simulink model "PubSub_Control_Thruster"  (R2018a)
settings: Solver=VariableStepAuto  StartTime=0.0  StopTime=inf  RelTol=1e-3
undefined symbols (not defined in the file or in its folder): angle_p_kp, angle_r_kp, angle_y_kp, Binv, Cx, Cy, DiscIntNeverNeededParam, Mx, My, omega_p_ki, omega_p_kp, omega_r_ki, omega_r_kp, omega_y_ki, omega_y_kp, RoboPlus_f2v_n, RoboPlus_f2v_p, Seabotix_f2v_n, Seabotix_f2v_p, serial, vx_kd, vx_ki, vx_kp, vy_kd, vy_ki, vy_kp, vz_ki, vz_kp, z_kp
libraries: simulink x10, robotlib x6, instrumentlib x2
settings Model: Creator=F.Takuya  LastModifiedBy=F.Takuya

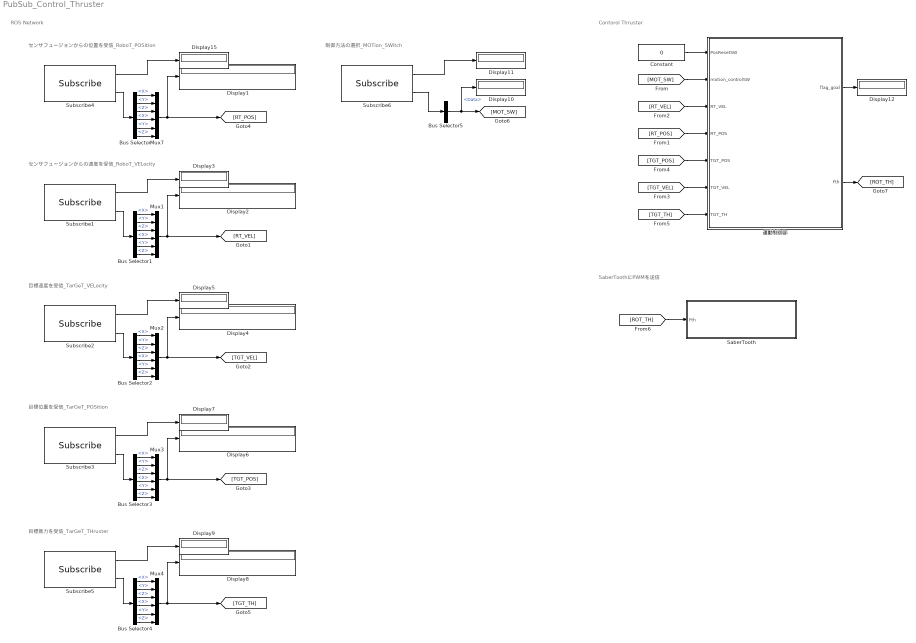
== system PubSub_Control_Thruster ==
  note: SaberToothにPWMを送信
  note: ROS Network
  note: センサフュージョンからの位置を受信_RoboT_POSition
  note: センサフュージョンからの速度を受信_RoboT_VELocity
  note: 目標速度を受信_TarGeT_VELocity
  note: 目標位置を受信_TarGeT_POSition
  note: 目標推力を受信_TarGeT_THruster
  note: 制御方法の選択_MOTion_SWitch
  note: Contorol Thruster
  Bus Selector{,1..4} (5 alike) : BusSelector  OutputSignals=Twist.Linear.X,Twist.Linear.Y,Twist.Linear.Z,Twist.Angular.X,Twist.Angular.Y,Twist.Angular.Z
  Bus Selector5 : BusSelector  OutputSignals=Data
  Constant : Constant  Value=0
  Display{1..12,15} (13 alike) : Display
  Mux{1..4,7} (5 alike) : Mux  Inputs=6
  SaberTooth : Subsystem
  Subscribe1 : robotlib/Subscribe  SourceLibraryInfo=This block requires Robotics System Toolbox  topicSource=Specify your own  topic=/RT_VEL  messageType=geometry_msgs/TwistStamped  sampleTime=-1  messageQueueLength=1
      settings: SourceProductBaseCode=RO
  Subscribe2 : robotlib/Subscribe  SourceLibraryInfo=This block requires Robotics System Toolbox  topicSource=Specify your own  topic=/TGT_VEL  messageType=geometry_msgs/TwistStamped  sampleTime=-1  messageQueueLength=1
      settings: SourceProductBaseCode=RO
  Subscribe3 : robotlib/Subscribe  SourceLibraryInfo=This block requires Robotics System Toolbox  topicSource=Specify your own  topic=/TGT_POS  messageType=geometry_msgs/TwistStamped  sampleTime=-1  messageQueueLength=1
      settings: SourceProductBaseCode=RO
  Subscribe4 : robotlib/Subscribe  SourceLibraryInfo=This block requires Robotics System Toolbox  topicSource=Specify your own  topic=/RT_POS  messageType=geometry_msgs/TwistStamped  sampleTime=-1  messageQueueLength=1
      settings: SourceProductBaseCode=RO
  Subscribe5 : robotlib/Subscribe  SourceLibraryInfo=This block requires Robotics System Toolbox  topicSource=Specify your own  topic=/TGT_TH  messageType=geometry_msgs/TwistStamped  sampleTime=-1  messageQueueLength=1
      settings: SourceProductBaseCode=RO
  Subscribe6 : robotlib/Subscribe  SourceLibraryInfo=This block requires Robotics System Toolbox  topicSource=Specify your own  topic=/MOT_SW  messageType=std_msgs/Float64  sampleTime=-1  messageQueueLength=1
      settings: SourceProductBaseCode=RO
  運動制御部 : Subsystem
  wires:
  Mux7/1 -> Display1/1, [RT_POS]
  Subscribe4/1 -> Display15/1
  Subscribe4/2 -> Bus Selector/1
  Bus Selector/1 -> Mux7/1  "<X>"
  Bus Selector/2 -> Mux7/2  "<Y>"
  Bus Selector/3 -> Mux7/3  "<Z>"
  Bus Selector/4 -> Mux7/4  "<X>"
  Bus Selector/5 -> Mux7/5  "<Y>"
  Bus Selector/6 -> Mux7/6  "<Z>"
  Subscribe1/2 -> Bus Selector1/1
  Bus Selector1/2 -> Mux1/2  "<Y>"
  Bus Selector1/1 -> Mux1/1  "<X>"
  Bus Selector1/5 -> Mux1/5  "<Y>"
  Mux1/1 -> Display2/1, [RT_VEL]
  Subscribe1/1 -> Display3/1
  Bus Selector1/4 -> Mux1/4  "<X>"
  Bus Selector1/3 -> Mux1/3  "<Z>"
  Bus Selector1/6 -> Mux1/6  "<Z>"
  Bus Selector2/3 -> Mux2/3  "<Z>"
  Subscribe2/1 -> Display5/1
  Bus Selector2/4 -> Mux2/4  "<X>"
  Bus Selector2/6 -> Mux2/6  "<Z>"
  Mux2/1 -> Display4/1, [TGT_VEL]
  Bus Selector2/5 -> Mux2/5  "<Y>"
  Bus Selector2/2 -> Mux2/2  "<Y>"
  Subscribe2/2 -> Bus Selector2/1
  Bus Selector2/1 -> Mux2/1  "<X>"
  Bus Selector3/4 -> Mux3/4  "<X>"
  Mux3/1 -> Display6/1, [TGT_POS]
  Bus Selector3/2 -> Mux3/2  "<Y>"
  Bus Selector3/1 -> Mux3/1  "<X>"
  Bus Selector3/5 -> Mux3/5  "<Y>"
  Bus Selector3/3 -> Mux3/3  "<Z>"
  Subscribe3/1 -> Display7/1
  Bus Selector3/6 -> Mux3/6  "<Z>"
  Subscribe3/2 -> Bus Selector3/1
  Subscribe5/2 -> Bus Selector4/1
  Subscribe5/1 -> Display9/1
  Bus Selector4/1 -> Mux4/1  "<X>"
  Bus Selector4/2 -> Mux4/2  "<Y>"
  Bus Selector4/6 -> Mux4/6  "<Z>"
  Bus Selector4/3 -> Mux4/3  "<Z>"
  Bus Selector4/4 -> Mux4/4  "<X>"
  Mux4/1 -> Display8/1, [TGT_TH]
  Bus Selector4/5 -> Mux4/5  "<Y>"
  Subscribe6/1 -> Display11/1
  Subscribe6/2 -> Bus Selector5/1
  Bus Selector5/1 -> Display10/1, [MOT_SW]  "<Data>"
  [TGT_TH] -> 運動制御部/7(TGT_TH)
  [TGT_VEL] -> 運動制御部/6(TGT_VEL)
  [TGT_POS] -> 運動制御部/5(TGT_POS)
  [RT_POS] -> 運動制御部/4(RT_POS)
  [RT_VEL] -> 運動制御部/3(RT_VEL)
  [MOT_SW] -> 運動制御部/2(motion_controlSW)
  運動制御部/2(Fth) -> [ROT_TH]
  運動制御部/1(flag_goal) -> Display12/1
  Constant/1 -> 運動制御部/1(PosResetSW)
  [ROT_TH] -> SaberTooth/1(Fth)

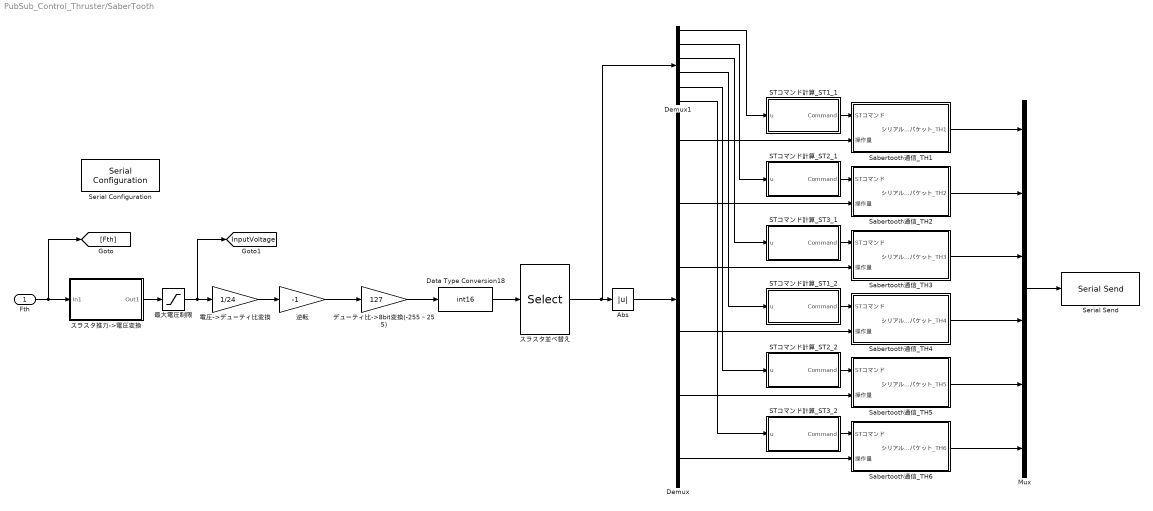
== system PubSub_Control_Thruster/SaberTooth ==
  Fth : Inport
  Abs : Abs
  Data Type Conversion18 : DataTypeConversion  OutDataTypeStr=int16
  Demux : Demux  Outputs=6
  Demux1 : Demux  Outputs=6
  Mux : Mux  Inputs=6
  STコマンド計算_ST1_1 : MATLAB Function  TreatAsAtomicUnit=on
  STコマンド計算_ST1_2 : MATLAB Function  TreatAsAtomicUnit=on
  STコマンド計算_ST2_1 : MATLAB Function  TreatAsAtomicUnit=on
  STコマンド計算_ST2_2 : MATLAB Function  TreatAsAtomicUnit=on
  STコマンド計算_ST3_1 : MATLAB Function  TreatAsAtomicUnit=on
  STコマンド計算_ST3_2 : MATLAB Function  TreatAsAtomicUnit=on
  Sabertooth通信_TH1 : Subsystem
  Sabertooth通信_TH2 : Subsystem
  Sabertooth通信_TH3 : Subsystem
  Sabertooth通信_TH4 : Subsystem
  Sabertooth通信_TH5 : Subsystem
  Sabertooth通信_TH6 : Subsystem
  Serial Configuration : instrumentlib/Serial Configuration  Priority=-200000  ComPortMenu=<Please select a port...>  ComPort=COM9  ObjConstructor=serial('COM9');  BaudRate=9600  DataBits=8  Parity=none  StopBits=1  FlowControl=none  Timeout=10  ByteOrder=LittleEndian
  Serial Send : instrumentlib/Serial Send  ComPortMenu=<Please select a port...>  ComPort=COM9  ObjConstructor=serial('COM9');  Terminator=<none>  EnableBlockingMode=on
  スラスタ並べ替え : Selector  InputPortWidth=6  IndexOptions=Index vector (dialog)  Indices=[4 5 1 6 3 2]  OutputSizes=1
  スラスタ推力->電圧変換 : Subsystem
  デューティ比->8bit変換(-255～255) : Gain  Gain=127
  最大電圧制限 : Saturate  UpperLimit=24  LowerLimit=-24
  逆転 : Gain  Gain=-1
  電圧->デューティ比変換 : Gain  Gain=1/24
  tag scope: InputVoltage=global
  wires:
  電圧->デューティ比変換/1 -> 逆転/1
  スラスタ推力->電圧変換/1(Out1) -> 最大電圧制限/1
  Fth/1 -> [Fth], スラスタ推力->電圧変換/1(In1)
  STコマンド計算_ST3_2/1(Command) -> Sabertooth通信_TH6/1(STコマンド)
  Sabertooth通信_TH4/1(シリアルパケット_TH4) -> Mux/4
  STコマンド計算_ST1_1/1(Command) -> Sabertooth通信_TH1/1(STコマンド)
  Sabertooth通信_TH1/1(シリアルパケット_TH1) -> Mux/1
  Mux/1 -> Serial Send/1
  Demux/3 -> Sabertooth通信_TH3/2(操作量)
  Sabertooth通信_TH5/1(シリアルパケット_TH5) -> Mux/5
  Demux/4 -> Sabertooth通信_TH4/2(操作量)
  Sabertooth通信_TH2/1(シリアルパケット_TH2) -> Mux/2
  Sabertooth通信_TH3/1(シリアルパケット_TH3) -> Mux/3
  Demux/1 -> Sabertooth通信_TH1/2(操作量)
  Sabertooth通信_TH6/1(シリアルパケット_TH6) -> Mux/6
  Demux/2 -> Sabertooth通信_TH2/2(操作量)
  Abs/1 -> Demux/1
  Demux/5 -> Sabertooth通信_TH5/2(操作量)
  Demux/6 -> Sabertooth通信_TH6/2(操作量)
  STコマンド計算_ST2_1/1(Command) -> Sabertooth通信_TH2/1(STコマンド)
  STコマンド計算_ST2_2/1(Command) -> Sabertooth通信_TH5/1(STコマンド)
  STコマンド計算_ST1_2/1(Command) -> Sabertooth通信_TH4/1(STコマンド)
  STコマンド計算_ST3_1/1(Command) -> Sabertooth通信_TH3/1(STコマンド)
  Demux1/6 -> STコマンド計算_ST3_2/1(u)
  Demux1/5 -> STコマンド計算_ST2_2/1(u)
  Demux1/4 -> STコマンド計算_ST1_2/1(u)
  Demux1/3 -> STコマンド計算_ST3_1/1(u)
  Demux1/2 -> STコマンド計算_ST2_1/1(u)
  Demux1/1 -> STコマンド計算_ST1_1/1(u)
  デューティ比->8bit変換(-255～255)/1 -> Data Type Conversion18/1
  Data Type Conversion18/1 -> スラスタ並べ替え/1
  スラスタ並べ替え/1 -> Abs/1, Demux1/1
  最大電圧制限/1 -> [InputVoltage], 電圧->デューティ比変換/1
  逆転/1 -> デューティ比->8bit変換(-255～255)/1

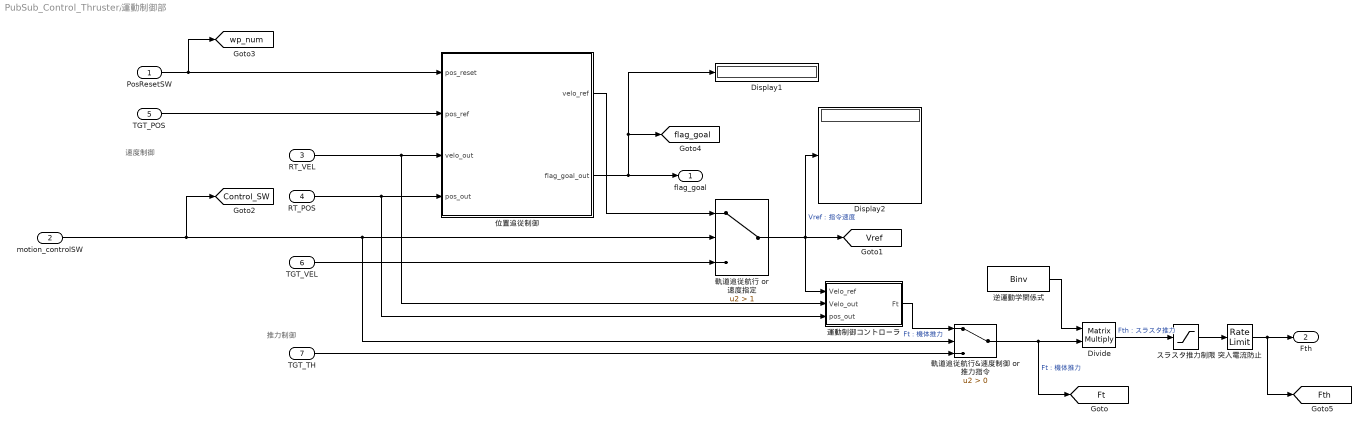
== system PubSub_Control_Thruster/運動制御部 ==
  note: 推力制御
  note: 速度制御
  PosResetSW : Inport
  motion_controlSW : Inport  Port=2
  RT_VEL : Inport  Port=3
  RT_POS : Inport  Port=4
  TGT_POS : Inport  Port=5
  TGT_VEL : Inport  Port=6
  TGT_TH : Inport  Port=7
  Display1 : Display
  Display2 : Display
  Divide : Product  Inputs=**  Multiplication=Matrix(*)
  スラスタ推力制限 : Saturate  UpperLimit=20  LowerLimit=-20
  位置追従制御 : Stateflow chart  TreatAsAtomicUnit=on
  突入電流防止 : RateLimiter  RisingSlewLimit=50  FallingSlewLimit=-50  SampleTimeMode=inherited
  軌道追従航行 or 速度指定 : Switch  Criteria=u2 > Threshold  Threshold=1
  軌道追従航行&速度制御 or 推力指令 : Switch  Criteria=u2 > Threshold
  逆運動学関係式 : Constant  Value=Binv
  運動制御コントローラ : Subsystem
  flag_goal : Outport
  Fth : Outport  Port=2
  tag scope: Control_SW=global, Ft=global, Fth=global, Vref=global, flag_goal=global, wp_num=global
  wires:
  軌道追従航行&速度制御 or 推力指令/1 -> [Ft], Divide/2  "Ft : 機体推力"
  軌道追従航行 or 速度指定/1 -> 運動制御コントローラ/1(Velo_ref), Display2/1, [Vref]  "Vref : 指令速度"
  逆運動学関係式/1 -> Divide/1
  Divide/1 -> スラスタ推力制限/1  "Fth : スラスタ推力"
  motion_controlSW/1 -> [Control_SW], 軌道追従航行&速度制御 or 推力指令/2, 軌道追従航行 or 速度指定/2
  TGT_VEL/1 -> 軌道追従航行 or 速度指定/3
  RT_VEL/1 -> 運動制御コントローラ/2(Velo_out), 位置追従制御/3(velo_out)
  運動制御コントローラ/1(Ft) -> 軌道追従航行&速度制御 or 推力指令/1  "Ft : 機体推力"
  RT_POS/1 -> 運動制御コントローラ/3(pos_out), 位置追従制御/4(pos_out)
  PosResetSW/1 -> 位置追従制御/1(pos_reset), [wp_num]
  位置追従制御/1(velo_ref) -> 軌道追従航行 or 速度指定/1
  TGT_TH/1 -> 軌道追従航行&速度制御 or 推力指令/3
  スラスタ推力制限/1 -> 突入電流防止/1
  突入電流防止/1 -> [Fth], Fth/1
  位置追従制御/2(flag_goal_out) -> Display1/1, [flag_goal], flag_goal/1
  TGT_POS/1 -> 位置追従制御/2(pos_ref)

== system PubSub_Control_Thruster/SaberTooth/Sabertooth通信_TH1 ==
  STコマンド : Inport
  操作量 : Inport  Port=2
  Add : Sum  Inputs=+++
  Address : Constant  Value=128  OutDataTypeStr=uint8
  Bitwise Operator : simulink/Logic and Bit Operations/Bitwise Operator  logicop=AND  UseBitMask=on  BitMask=bin2dec('01111111')  BitMaskRealWorld=Stored Integer
  Data Type Conversion{,1..3} (4 alike) : DataTypeConversion  OutDataTypeStr=uint8
  Mux : Mux
  Saturation : Saturate  UpperLimit=255  LowerLimit=0
  Saturation1 : Saturate  UpperLimit=255  LowerLimit=0
  Scope : Scope
  シリアルパケット_TH1 : Outport
  wires:
  Bitwise Operator/1 -> Mux/4  "チェックサム address byte  + command byte  + data byte"
  Data Type Conversion2/1 -> Saturation1/1
  Data Type Conversion1/1 -> Bitwise Operator/1
  STコマンド/1 -> Data Type Conversion3/1  "コマンド [モーター１] 0：正転　1：逆転 [モーター2] 4：正転　5：逆転"
  操作量/1 -> Data Type Conversion2/1
  Mux/1 -> Saturation/1
  Data Type Conversion/1 -> シリアルパケット_TH1/1
  Add/1 -> Data Type Conversion1/1
  Saturation/1 -> Data Type Conversion/1
  Address/1 -> Add/1, Mux/1  "Sabertoothのアドレス（どのSTと通信するか）"
  Saturation1/1 -> Scope/1, Add/3, Mux/3  "操作量(uint8の0～255)"
  Data Type Conversion3/1 -> Add/2, Mux/2

== system PubSub_Control_Thruster/SaberTooth/Sabertooth通信_TH2 ==
  STコマンド : Inport
  操作量 : Inport  Port=2
  Add : Sum  Inputs=+++
  Address : Constant  Value=129  OutDataTypeStr=uint8
  Bitwise Operator : simulink/Logic and Bit Operations/Bitwise Operator  logicop=AND  UseBitMask=on  BitMask=bin2dec('01111111')  BitMaskRealWorld=Stored Integer
  Data Type Conversion{,1..3} (4 alike) : DataTypeConversion  OutDataTypeStr=uint8
  Mux : Mux
  Saturation : Saturate  UpperLimit=255  LowerLimit=0
  Saturation1 : Saturate  UpperLimit=255  LowerLimit=0
  Scope : Scope
  シリアルパケット_TH2 : Outport
  wires:
  Bitwise Operator/1 -> Mux/4  "チェックサム address byte  + command byte  + data byte"
  Data Type Conversion2/1 -> Saturation1/1
  Data Type Conversion1/1 -> Bitwise Operator/1
  STコマンド/1 -> Data Type Conversion3/1  "コマンド [モーター１] 0：正転　1：逆転 [モーター2] 4：正転　5：逆転"
  操作量/1 -> Data Type Conversion2/1
  Mux/1 -> Saturation/1
  Data Type Conversion/1 -> シリアルパケット_TH2/1
  Add/1 -> Data Type Conversion1/1
  Saturation/1 -> Data Type Conversion/1
  Address/1 -> Add/1, Mux/1  "Sabertoothのアドレス（どのSTと通信するか）"
  Saturation1/1 -> Scope/1, Add/3, Mux/3  "操作量(uint8の0～255)"
  Data Type Conversion3/1 -> Add/2, Mux/2

== system PubSub_Control_Thruster/SaberTooth/Sabertooth通信_TH3 ==
  STコマンド : Inport
  操作量 : Inport  Port=2
  Add : Sum  Inputs=+++
  Address : Constant  Value=130  OutDataTypeStr=uint8
  Bitwise Operator : simulink/Logic and Bit Operations/Bitwise Operator  logicop=AND  UseBitMask=on  BitMask=bin2dec('01111111')  BitMaskRealWorld=Stored Integer
  Data Type Conversion{,1..3} (4 alike) : DataTypeConversion  OutDataTypeStr=uint8
  Mux : Mux
  Saturation : Saturate  UpperLimit=255  LowerLimit=0
  Saturation1 : Saturate  UpperLimit=255  LowerLimit=0
  Scope : Scope
  シリアルパケット_TH3 : Outport
  wires:
  Bitwise Operator/1 -> Mux/4  "チェックサム address byte  + command byte  + data byte"
  Data Type Conversion2/1 -> Saturation1/1
  Data Type Conversion1/1 -> Bitwise Operator/1
  STコマンド/1 -> Data Type Conversion3/1  "コマンド [モーター１] 0：正転　1：逆転 [モーター2] 4：正転　5：逆転"
  操作量/1 -> Data Type Conversion2/1
  Mux/1 -> Saturation/1
  Data Type Conversion/1 -> シリアルパケット_TH3/1
  Add/1 -> Data Type Conversion1/1
  Saturation/1 -> Data Type Conversion/1
  Address/1 -> Add/1, Mux/1  "Sabertoothのアドレス（どのSTと通信するか）"
  Saturation1/1 -> Scope/1, Add/3, Mux/3  "操作量(uint8の0～255)"
  Data Type Conversion3/1 -> Add/2, Mux/2

== system PubSub_Control_Thruster/SaberTooth/Sabertooth通信_TH4 ==
  STコマンド : Inport
  操作量 : Inport  Port=2
  Add : Sum  Inputs=+++
  Address : Constant  Value=128  OutDataTypeStr=uint8
  Bitwise Operator : simulink/Logic and Bit Operations/Bitwise Operator  logicop=AND  UseBitMask=on  BitMask=bin2dec('01111111')  BitMaskRealWorld=Stored Integer
  Data Type Conversion{,1..3} (4 alike) : DataTypeConversion  OutDataTypeStr=uint8
  Mux : Mux
  Saturation : Saturate  UpperLimit=255  LowerLimit=0
  Saturation1 : Saturate  UpperLimit=255  LowerLimit=0
  Scope : Scope
  シリアルパケット_TH4 : Outport
  wires:
  Bitwise Operator/1 -> Mux/4  "チェックサム address byte  + command byte  + data byte"
  Data Type Conversion2/1 -> Saturation1/1
  Data Type Conversion1/1 -> Bitwise Operator/1
  STコマンド/1 -> Data Type Conversion3/1  "コマンド [モーター１] 0：正転　1：逆転 [モーター2] 4：正転　5：逆転"
  操作量/1 -> Data Type Conversion2/1
  Mux/1 -> Saturation/1
  Data Type Conversion/1 -> シリアルパケット_TH4/1
  Add/1 -> Data Type Conversion1/1
  Saturation/1 -> Data Type Conversion/1
  Address/1 -> Add/1, Mux/1  "Sabertoothのアドレス（どのSTと通信するか）"
  Saturation1/1 -> Scope/1, Add/3, Mux/3  "操作量(uint8の0～255)"
  Data Type Conversion3/1 -> Add/2, Mux/2

== system PubSub_Control_Thruster/SaberTooth/Sabertooth通信_TH5 ==
  STコマンド : Inport
  操作量 : Inport  Port=2
  Add : Sum  Inputs=+++
  Address : Constant  Value=129  OutDataTypeStr=uint8
  Bitwise Operator : simulink/Logic and Bit Operations/Bitwise Operator  logicop=AND  UseBitMask=on  BitMask=bin2dec('01111111')  BitMaskRealWorld=Stored Integer
  Data Type Conversion{,1..3} (4 alike) : DataTypeConversion  OutDataTypeStr=uint8
  Mux : Mux
  Saturation : Saturate  UpperLimit=255  LowerLimit=0
  Saturation1 : Saturate  UpperLimit=255  LowerLimit=0
  Scope : Scope
  シリアルパケット_TH5 : Outport
  wires:
  Bitwise Operator/1 -> Mux/4  "チェックサム address byte  + command byte  + data byte"
  Data Type Conversion2/1 -> Saturation1/1
  Data Type Conversion1/1 -> Bitwise Operator/1
  STコマンド/1 -> Data Type Conversion3/1  "コマンド [モーター１] 0：正転　1：逆転 [モーター2] 4：正転　5：逆転"
  操作量/1 -> Data Type Conversion2/1
  Mux/1 -> Saturation/1
  Data Type Conversion/1 -> シリアルパケット_TH5/1
  Add/1 -> Data Type Conversion1/1
  Saturation/1 -> Data Type Conversion/1
  Address/1 -> Add/1, Mux/1  "Sabertoothのアドレス（どのSTと通信するか）"
  Saturation1/1 -> Scope/1, Add/3, Mux/3  "操作量(uint8の0～255)"
  Data Type Conversion3/1 -> Add/2, Mux/2

== system PubSub_Control_Thruster/SaberTooth/Sabertooth通信_TH6 ==
  STコマンド : Inport
  操作量 : Inport  Port=2
  Add : Sum  Inputs=+++
  Address : Constant  Value=130  OutDataTypeStr=uint8
  Bitwise Operator : simulink/Logic and Bit Operations/Bitwise Operator  logicop=AND  UseBitMask=on  BitMask=bin2dec('01111111')  BitMaskRealWorld=Stored Integer
  Data Type Conversion{,1..3} (4 alike) : DataTypeConversion  OutDataTypeStr=uint8
  Mux : Mux
  Saturation : Saturate  UpperLimit=255  LowerLimit=0
  Saturation1 : Saturate  UpperLimit=255  LowerLimit=0
  Scope : Scope
  シリアルパケット_TH6 : Outport
  wires:
  Bitwise Operator/1 -> Mux/4  "チェックサム address byte  + command byte  + data byte"
  Data Type Conversion2/1 -> Saturation1/1
  Data Type Conversion1/1 -> Bitwise Operator/1
  STコマンド/1 -> Data Type Conversion3/1  "コマンド [モーター１] 0：正転　1：逆転 [モーター2] 4：正転　5：逆転"
  操作量/1 -> Data Type Conversion2/1
  Mux/1 -> Saturation/1
  Data Type Conversion/1 -> シリアルパケット_TH6/1
  Add/1 -> Data Type Conversion1/1
  Saturation/1 -> Data Type Conversion/1
  Address/1 -> Add/1, Mux/1  "Sabertoothのアドレス（どのSTと通信するか）"
  Saturation1/1 -> Scope/1, Add/3, Mux/3  "操作量(uint8の0～255)"
  Data Type Conversion3/1 -> Add/2, Mux/2

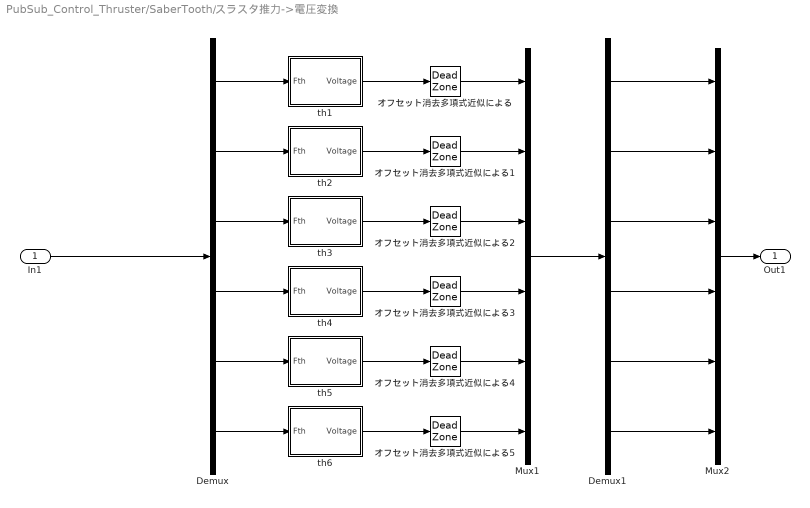
== system PubSub_Control_Thruster/SaberTooth/スラスタ推力->電圧変換 ==
  In1 : Inport
  Demux : Demux  Outputs=6
  Demux1 : Demux  Outputs=6
  Mux1 : Mux  Inputs=6
  Mux2 : Mux  Inputs=6
  th1 : Subsystem
  th2 : Subsystem
  th3 : Subsystem
  th4 : Subsystem
  th5 : Subsystem
  th6 : Subsystem
  オフセット消去多項式近似による{,1,4..5} (4 alike) : DeadZone  LowerValue=Seabotix_f2v_n(4)  UpperValue=Seabotix_f2v_p(4)  SaturateOnIntegerOverflow=on
  オフセット消去多項式近似による2 : DeadZone  LowerValue=RoboPlus_f2v_n(4)  UpperValue=RoboPlus_f2v_p(4)  SaturateOnIntegerOverflow=on
  オフセット消去多項式近似による3 : DeadZone  LowerValue=RoboPlus_f2v_n(4)  UpperValue=RoboPlus_f2v_p(4)  SaturateOnIntegerOverflow=on
  Out1 : Outport
  wires:
  th1/1(Voltage) -> オフセット消去多項式近似による/1
  Demux/1 -> th1/1(Fth)
  Demux/2 -> th2/1(Fth)
  th4/1(Voltage) -> オフセット消去多項式近似による3/1
  Demux/3 -> th3/1(Fth)
  th3/1(Voltage) -> オフセット消去多項式近似による2/1
  Demux/4 -> th4/1(Fth)
  Mux1/1 -> Demux1/1
  Demux1/5 -> Mux2/5
  Demux1/6 -> Mux2/6
  Demux1/4 -> Mux2/4
  Demux1/3 -> Mux2/3
  Demux1/2 -> Mux2/2
  Demux1/1 -> Mux2/1
  Mux2/1 -> Out1/1
  オフセット消去多項式近似による/1 -> Mux1/1
  オフセット消去多項式近似による2/1 -> Mux1/3
  オフセット消去多項式近似による3/1 -> Mux1/4
  オフセット消去多項式近似による4/1 -> Mux1/5
  Demux/6 -> th6/1(Fth)
  Demux/5 -> th5/1(Fth)
  In1/1 -> Demux/1
  th2/1(Voltage) -> オフセット消去多項式近似による1/1
  オフセット消去多項式近似による1/1 -> Mux1/2
  th5/1(Voltage) -> オフセット消去多項式近似による4/1
  th6/1(Voltage) -> オフセット消去多項式近似による5/1
  オフセット消去多項式近似による5/1 -> Mux1/6

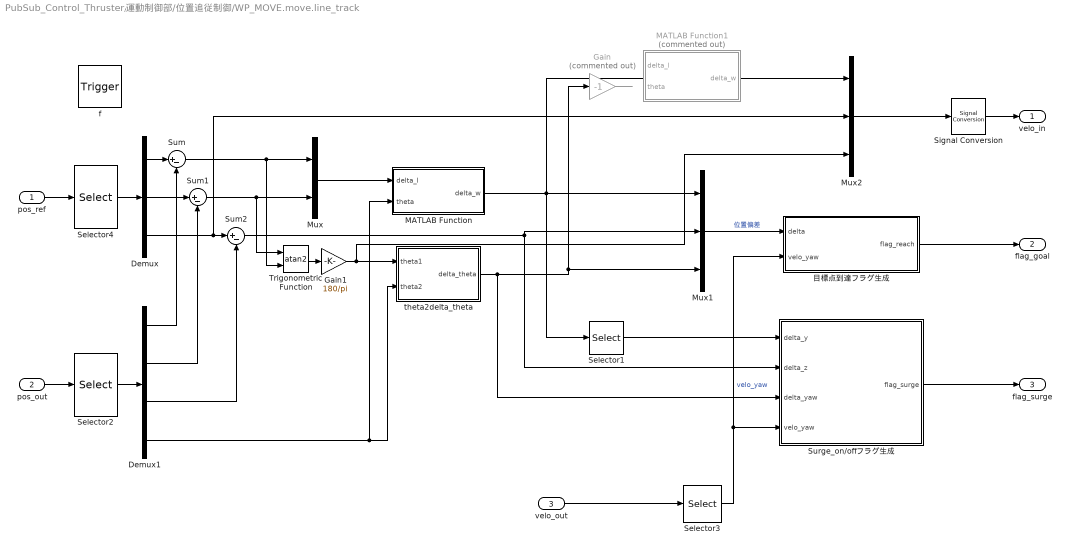
== system PubSub_Control_Thruster/運動制御部/位置追従制御/WP_MOVE.move.line_track ==
  pos_ref : Inport  OutDataTypeStr=double  PortDimensions=6
  pos_out : Inport  Port=2  OutDataTypeStr=double  PortDimensions=6
  velo_out : Inport  Port=3  OutDataTypeStr=double  PortDimensions=6
  f : TriggerPort  TriggerType=function-call  VariantControl=Variant
      settings: CopyFcn=Stateflow.SLINSF.SimulinkMan.removeBlockPreDeleteFcn  PreDeleteFcn=Stateflow.SLINSF.SimulinkMan.unsafePredeleteFcn
  Demux : Demux  Outputs=3
  Demux1 : Demux
  Gain : Gain  Commented=on  Gain=-1
  Gain1 : Gain  Gain=180/pi
  MATLAB Function : MATLAB Function  TreatAsAtomicUnit=on
  MATLAB Function1 : MATLAB Function  Commented=on  TreatAsAtomicUnit=on
  Mux : Mux  Inputs=2
  Mux1 : Mux  Inputs=3
  Mux2 : Mux  Inputs=3
  Selector1 : Selector  InputPortWidth=2  IndexOptions=Index vector (dialog)  Indices=[2]  OutputSizes=1
  Selector2 : Selector  InputPortWidth=6  IndexOptions=Index vector (dialog)  Indices=[1 2 3 6]  OutputSizes=1
  Selector3 : Selector  InputPortWidth=6  IndexOptions=Index vector (dialog)  Indices=[6]  OutputSizes=1
  Selector4 : Selector  InputPortWidth=6  IndexOptions=Index vector (dialog)  Indices=[1 2 3 ]  OutputSizes=1
  Signal Conversion : SignalConversion  OverrideOpt=off
  Sum : Sum  Inputs=|+-
  Sum1 : Sum  Inputs=|+-
  Sum2 : Sum  Inputs=|+-
  Surge_on/offフラグ生成 : MATLAB Function  TreatAsAtomicUnit=on
  Trigonometric Function : Trigonometry  Operator=atan2
  theta2delta_theta : Subsystem
  目標点到達フラグ生成 : MATLAB Function  TreatAsAtomicUnit=on
  velo_in : Outport  OutDataTypeStr=double  PortDimensions=4
  flag_goal : Outport  Port=2  OutDataTypeStr=double  PortDimensions=1
  flag_surge : Outport  Port=3  OutDataTypeStr=double  PortDimensions=1
  wires:
  pos_ref/1 -> Selector4/1
  pos_out/1 -> Selector2/1
  Mux/1 -> MATLAB Function/1(delta_l)
  Sum/1 -> Trigonometric Function/2, Mux/1
  Demux/1 -> Sum/1
  Demux1/1 -> Sum/2
  Sum1/1 -> Trigonometric Function/1, Mux/2
  Demux/2 -> Sum1/1
  Demux1/2 -> Sum1/2
  Demux1/3 -> Sum2/2
  Sum2/1 -> Surge_on/offフラグ生成/2(delta_z), Mux1/2
  theta2delta_theta/1(delta_theta) -> Surge_on/offフラグ生成/3(delta_yaw), Gain/1, Mux1/3
  Mux2/1 -> Signal Conversion/1
  Selector1/1 -> Surge_on/offフラグ生成/1(delta_y)
  MATLAB Function/1(delta_w) -> Selector1/1, Mux1/1, Mux2/1
  目標点到達フラグ生成/1(flag_reach) -> flag_goal/1
  Surge_on/offフラグ生成/1(flag_surge) -> flag_surge/1
  Selector2/1 -> Demux1/1
  Mux1/1 -> 目標点到達フラグ生成/1(delta)  "位置偏差"
  Demux/3 -> Mux2/2, Sum2/1
  Demux1/4 -> MATLAB Function/2(theta), theta2delta_theta/2(theta2)
  Gain/1 -> ?
  velo_out/1 -> Selector3/1
  Selector3/1 -> 目標点到達フラグ生成/2(velo_yaw), Surge_on/offフラグ生成/4(velo_yaw)  "velo_yaw"
  Signal Conversion/1 -> velo_in/1
  Selector4/1 -> Demux/1
  Trigonometric Function/1 -> Gain1/1
  Gain1/1 -> Mux2/3, theta2delta_theta/1(theta1)

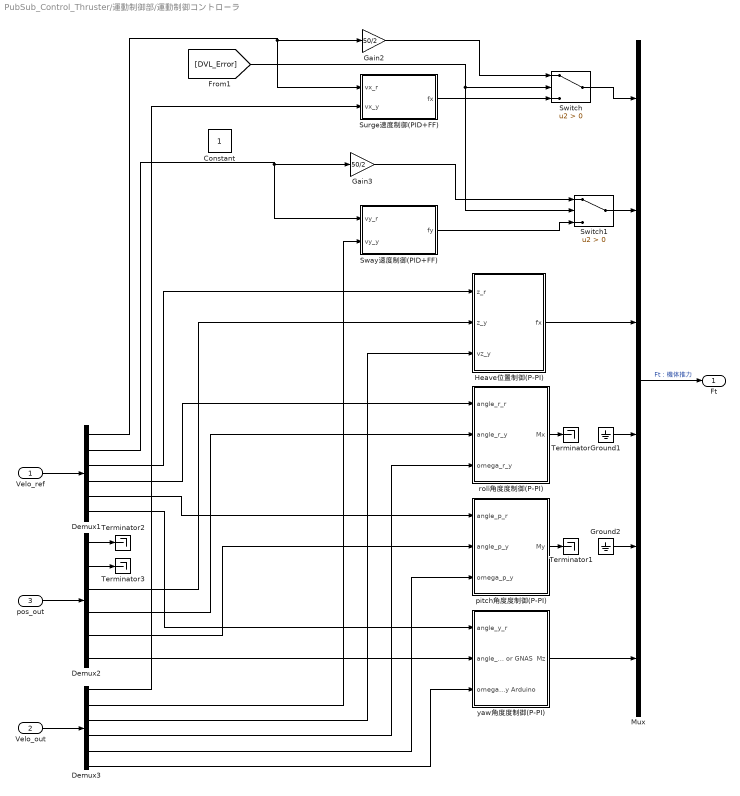
== system PubSub_Control_Thruster/運動制御部/運動制御コントローラ ==
  Velo_ref : Inport
  Velo_out : Inport  Port=2
  pos_out : Inport  Port=3
  Constant : Constant
  Demux1 : Demux  Outputs=6
  Demux2 : Demux  Outputs=6
  Demux3 : Demux  Outputs=6
  Gain2 : Gain  Gain=50/2
  Gain3 : Gain  Gain=50/2
  Ground1 : Ground
  Ground2 : Ground
  Heave位置制御(P-PI) : Subsystem
  Mux : Mux  Inputs=6
  Surge速度制御(PID+FF) : Subsystem
  Sway速度制御(PID+FF) : Subsystem
  Switch : Switch  Criteria=u2 > Threshold
  Switch1 : Switch  Criteria=u2 > Threshold
  Terminator{,1..3} (4 alike) : Terminator
  pitch角度度制御(P-PI) : Subsystem
  roll角度度制御(P-PI) : Subsystem
  yaw角度度制御(P-PI) : Subsystem
  Ft : Outport
  wires:
  Demux1/1 -> Surge速度制御(PID+FF)/1(vx_r), Gain2/1
  yaw角度度制御(P-PI)/1(Mz) -> Mux/6
  Demux1/2 -> Sway速度制御(PID+FF)/1(vy_r), Gain3/1
  Switch1/1 -> Mux/2
  Sway速度制御(PID+FF)/1(fy) -> Switch1/3
  Switch/1 -> Mux/1
  [DVL_Error] -> Switch/2, Switch1/2
  Surge速度制御(PID+FF)/1(fx) -> Switch/3
  Demux3/1 -> Surge速度制御(PID+FF)/2(vx_y)
  Heave位置制御(P-PI)/1(fx) -> Mux/3
  Velo_out/1 -> Demux3/1
  Demux2/1 -> Terminator2/1
  Demux2/2 -> Terminator3/1
  pos_out/1 -> Demux2/1
  pitch角度度制御(P-PI)/1(My) -> Terminator1/1
  roll角度度制御(P-PI)/1(Mx) -> Terminator/1
  Ground2/1 -> Mux/5
  Demux2/4 -> roll角度度制御(P-PI)/2(angle_r_y)
  Demux3/4 -> roll角度度制御(P-PI)/3(omega_r_y)
  Demux1/4 -> roll角度度制御(P-PI)/1(angle_r_r)
  Demux2/5 -> pitch角度度制御(P-PI)/2(angle_p_y)
  Demux3/5 -> pitch角度度制御(P-PI)/3(omega_p_y)
  Demux1/5 -> pitch角度度制御(P-PI)/1(angle_p_r)
  Ground1/1 -> Mux/4
  Demux3/3 -> Heave位置制御(P-PI)/3(vz_y)
  Demux2/6 -> yaw角度度制御(P-PI)/2(angle_y_y Arduiono or trax or GNAS)
  Demux3/2 -> Sway速度制御(PID+FF)/2(vy_y)
  Demux2/3 -> Heave位置制御(P-PI)/2(z_y)
  Demux3/6 -> yaw角度度制御(P-PI)/3(omega_y_y Arduino)
  Velo_ref/1 -> Demux1/1
  Demux1/6 -> yaw角度度制御(P-PI)/1(angle_y_r)
  Demux1/3 -> Heave位置制御(P-PI)/1(z_r)
  Mux/1 -> Ft/1  "Ft : 機体推力"
  Gain2/1 -> Switch/1
  Gain3/1 -> Switch1/1

== system PubSub_Control_Thruster/SaberTooth/スラスタ推力->電圧変換/th1 ==
  Fth : Inport
  Switch : Switch
  スラスタ推力->電圧 (F<0) : Fcn  Expr=(Seabotix_f2v_n(1)*u^3) + (Seabotix_f2v_n(2)*u^2) + (Seabotix_f2v_n(3)*u) + Seabotix_f2v_n(4)
  スラスタ推力->電圧 (F>=0) : Fcn  Expr=(Seabotix_f2v_p(1)*u^3) + (Seabotix_f2v_p(2)*u^2) + (Seabotix_f2v_p(3)*u) + Seabotix_f2v_p(4)
  Voltage : Outport
  wires:
  Switch/1 -> Voltage/1
  Fth/1 -> スラスタ推力->電圧 (F<0)/1, スラスタ推力->電圧 (F>=0)/1, Switch/2
  スラスタ推力->電圧 (F<0)/1 -> Switch/3
  スラスタ推力->電圧 (F>=0)/1 -> Switch/1

== system PubSub_Control_Thruster/SaberTooth/スラスタ推力->電圧変換/th2 ==
  Fth : Inport
  Switch : Switch
  スラスタ推力->電圧 (F<0) : Fcn  Expr=(Seabotix_f2v_n(1)*u^3) + (Seabotix_f2v_n(2)*u^2) + (Seabotix_f2v_n(3)*u) + Seabotix_f2v_n(4)
  スラスタ推力->電圧 (F>=0) : Fcn  Expr=(Seabotix_f2v_p(1)*u^3) + (Seabotix_f2v_p(2)*u^2) + (Seabotix_f2v_p(3)*u) + Seabotix_f2v_p(4)
  Voltage : Outport
  wires:
  Switch/1 -> Voltage/1
  Fth/1 -> スラスタ推力->電圧 (F<0)/1, スラスタ推力->電圧 (F>=0)/1, Switch/2
  スラスタ推力->電圧 (F<0)/1 -> Switch/3
  スラスタ推力->電圧 (F>=0)/1 -> Switch/1

== system PubSub_Control_Thruster/SaberTooth/スラスタ推力->電圧変換/th3 ==
  Fth : Inport
  Switch : Switch
  スラスタ推力->電圧 (F<0) : Fcn  Expr=(RoboPlus_f2v_n(1)*u^3) + (RoboPlus_f2v_n(2)*u^2) + (RoboPlus_f2v_n(3)*u) + RoboPlus_f2v_n(4)
  スラスタ推力->電圧 (F>=0) : Fcn  Expr=(RoboPlus_f2v_p(1)*u^3) + (RoboPlus_f2v_p(2)*u^2) + (RoboPlus_f2v_p(3)*u) + RoboPlus_f2v_p(4)
  Voltage : Outport
  wires:
  Switch/1 -> Voltage/1
  Fth/1 -> スラスタ推力->電圧 (F<0)/1, スラスタ推力->電圧 (F>=0)/1, Switch/2
  スラスタ推力->電圧 (F<0)/1 -> Switch/3
  スラスタ推力->電圧 (F>=0)/1 -> Switch/1

== system PubSub_Control_Thruster/SaberTooth/スラスタ推力->電圧変換/th4 ==
  Fth : Inport
  Switch : Switch
  スラスタ推力->電圧 (F<0) : Fcn  Expr=(RoboPlus_f2v_n(1)*u^3) + (RoboPlus_f2v_n(2)*u^2) + (RoboPlus_f2v_n(3)*u) + RoboPlus_f2v_n(4)
  スラスタ推力->電圧 (F>=0) : Fcn  Expr=(RoboPlus_f2v_p(1)*u^3) + (RoboPlus_f2v_p(2)*u^2) + (RoboPlus_f2v_p(3)*u) + RoboPlus_f2v_p(4)
  Voltage : Outport
  wires:
  Switch/1 -> Voltage/1
  Fth/1 -> スラスタ推力->電圧 (F<0)/1, スラスタ推力->電圧 (F>=0)/1, Switch/2
  スラスタ推力->電圧 (F<0)/1 -> Switch/3
  スラスタ推力->電圧 (F>=0)/1 -> Switch/1

== system PubSub_Control_Thruster/SaberTooth/スラスタ推力->電圧変換/th5 ==
  Fth : Inport
  Switch : Switch
  スラスタ推力->電圧 (F<0) : Fcn  Expr=(Seabotix_f2v_n(1)*u^3) + (Seabotix_f2v_n(2)*u^2) + (Seabotix_f2v_n(3)*u) + Seabotix_f2v_n(4)
  スラスタ推力->電圧 (F>=0) : Fcn  Expr=(Seabotix_f2v_p(1)*u^3) + (Seabotix_f2v_p(2)*u^2) + (Seabotix_f2v_p(3)*u) + Seabotix_f2v_p(4)
  Voltage : Outport
  wires:
  スラスタ推力->電圧 (F>=0)/1 -> Switch/1
  スラスタ推力->電圧 (F<0)/1 -> Switch/3
  Fth/1 -> Switch/2, スラスタ推力->電圧 (F>=0)/1, スラスタ推力->電圧 (F<0)/1
  Switch/1 -> Voltage/1

== system PubSub_Control_Thruster/SaberTooth/スラスタ推力->電圧変換/th6 ==
  Fth : Inport
  Switch : Switch
  スラスタ推力->電圧 (F<0) : Fcn  Expr=(Seabotix_f2v_n(1)*u^3) + (Seabotix_f2v_n(2)*u^2) + (Seabotix_f2v_n(3)*u) + Seabotix_f2v_n(4)
  スラスタ推力->電圧 (F>=0) : Fcn  Expr=(Seabotix_f2v_p(1)*u^3) + (Seabotix_f2v_p(2)*u^2) + (Seabotix_f2v_p(3)*u) + Seabotix_f2v_p(4)
  Voltage : Outport
  wires:
  Switch/1 -> Voltage/1
  Fth/1 -> スラスタ推力->電圧 (F<0)/1, スラスタ推力->電圧 (F>=0)/1, Switch/2
  スラスタ推力->電圧 (F<0)/1 -> Switch/3
  スラスタ推力->電圧 (F>=0)/1 -> Switch/1

== system PubSub_Control_Thruster/運動制御部/位置追従制御/WP_MOVE.move.line_track/theta2delta_theta ==
  theta1 : Inport
  theta2 : Inport  Port=2
  MATLAB Function : MATLAB Function  TreatAsAtomicUnit=on
  MATLAB Function1 : MATLAB Function  TreatAsAtomicUnit=on
  MATLAB Function2 : MATLAB Function  TreatAsAtomicUnit=on
  Sum : Sum  Inputs=|+-
  delta_theta : Outport
  wires:
  theta2/1 -> MATLAB Function1/1(theta_in)
  theta1/1 -> MATLAB Function/1(theta_in)
  MATLAB Function2/1(theta_out) -> delta_theta/1
  MATLAB Function/1(theta_out) -> Sum/1
  MATLAB Function1/1(theta_out) -> Sum/2
  Sum/1 -> MATLAB Function2/1(theta_in)

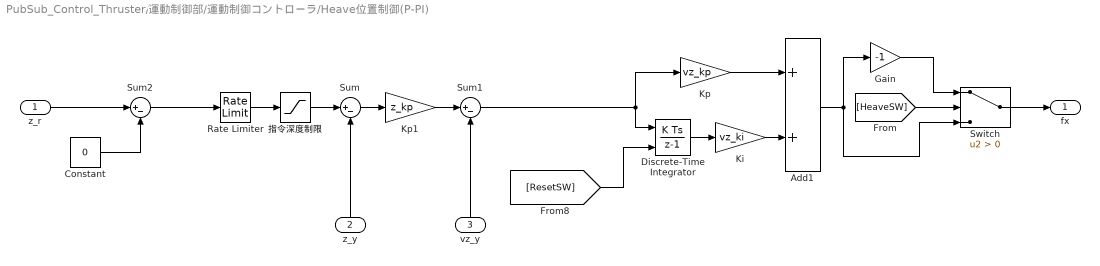
== system PubSub_Control_Thruster/運動制御部/運動制御コントローラ/Heave位置制御(P-PI) ==
  z_r : Inport
  z_y : Inport  Port=2
  vz_y : Inport  Port=3
  Add1 : Sum
  Constant : Constant  Value=0
  Discrete-Time Integrator : DiscreteIntegrator  ExternalReset=rising  SampleTime=-1  ICPrevOutput=DiscIntNeverNeededParam  ICPrevScaledInput=DiscIntNeverNeededParam
  Gain : Gain  Gain=-1
  Ki : Gain  Gain=vz_ki
  Kp : Gain  Gain=vz_kp
  Kp1 : Gain  Gain=z_kp
  Rate Limiter : RateLimiter  RisingSlewLimit=0.25  FallingSlewLimit=-0.25  SampleTimeMode=inherited
  Sum : Sum  Inputs=|+-
  Sum1 : Sum  Inputs=|+-
  Sum2 : Sum  Inputs=|+-
  Switch : Switch  Criteria=u2 > Threshold
  指令深度制限 : Saturate  UpperLimit=50  LowerLimit=-1
  fx : Outport
  wires:
  Constant/1 -> Sum2/2
  Sum2/1 -> Rate Limiter/1
  Add1/1 -> Switch/3, Gain/1
  Gain/1 -> Switch/1
  [HeaveSW] -> Switch/2
  Switch/1 -> fx/1
  Rate Limiter/1 -> 指令深度制限/1
  Sum1/1 -> Kp/1, Discrete-Time Integrator/1
  vz_y/1 -> Sum1/2
  Kp1/1 -> Sum1/1
  Sum/1 -> Kp1/1
  z_y/1 -> Sum/2
  z_r/1 -> Sum2/1
  Kp/1 -> Add1/1
  Discrete-Time Integrator/1 -> Ki/1
  Ki/1 -> Add1/2
  指令深度制限/1 -> Sum/1
  [ResetSW] -> Discrete-Time Integrator/2

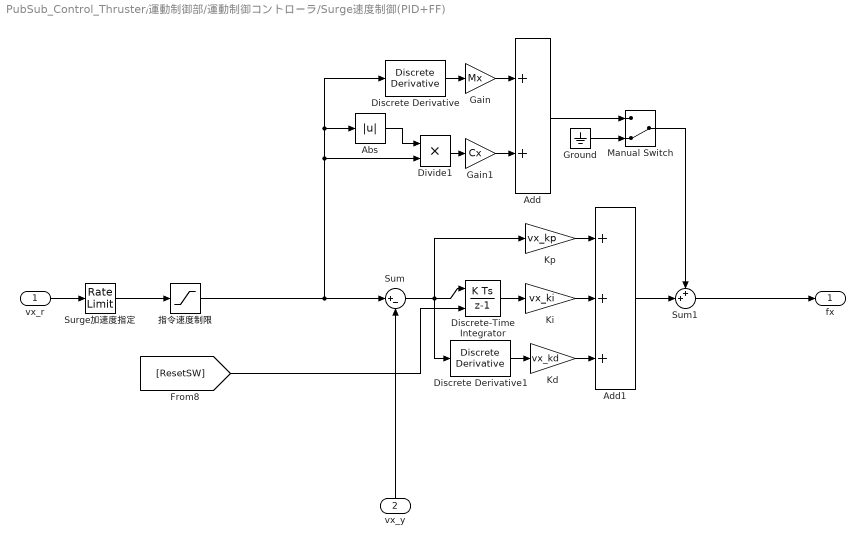
== system PubSub_Control_Thruster/運動制御部/運動制御コントローラ/Surge速度制御(PID+FF) ==
  vx_r : Inport
  vx_y : Inport  Port=2
  Abs : Abs
  Add : Sum
  Add1 : Sum  Inputs=+++
  Discrete Derivative : simulink/Discrete/Discrete Derivative  gainval=1.0  ICPrevScaledInput=0.0  InputProcessing=Inherited  OutMin=[]  OutMax=[]  OutDataType=fixdt(1, 16)  OutScaling=2^-10  DoSatur=off
  Discrete Derivative1 : simulink/Discrete/Discrete Derivative  gainval=1.0  ICPrevScaledInput=0.0  InputProcessing=Inherited  OutMin=[]  OutMax=[]  OutDataType=fixdt(1, 16)  OutScaling=2^-10  DoSatur=off
  Discrete-Time Integrator : DiscreteIntegrator  ExternalReset=rising  SampleTime=-1  ICPrevOutput=DiscIntNeverNeededParam  ICPrevScaledInput=DiscIntNeverNeededParam
  Divide1 : Product  Inputs=**
  Gain : Gain  Gain=Mx
  Gain1 : Gain  Gain=Cx
  Ground : Ground
  Kd : Gain  Gain=vx_kd
  Ki : Gain  Gain=vx_ki
  Kp : Gain  Gain=vx_kp
  Manual Switch : ManualSwitch  CurrentSetting=0
  Sum : Sum  Inputs=|+-
  Sum1 : Sum  Inputs=++|
  Surge加速度指定 : RateLimiter  RisingSlewLimit=0.3  FallingSlewLimit=-0.3  SampleTimeMode=inherited
  指令速度制限 : Saturate
  fx : Outport
  wires:
  Surge加速度指定/1 -> 指令速度制限/1
  Ground/1 -> Manual Switch/2
  Manual Switch/1 -> Sum1/1
  Add/1 -> Manual Switch/1
  vx_y/1 -> Sum/2
  vx_r/1 -> Surge加速度指定/1
  Kp/1 -> Add1/1
  Sum1/1 -> fx/1
  Discrete-Time Integrator/1 -> Ki/1
  Ki/1 -> Add1/2
  Sum/1 -> Discrete-Time Integrator/1, Kp/1, Discrete Derivative1/1
  Discrete Derivative1/1 -> Kd/1
  指令速度制限/1 -> Abs/1, Discrete Derivative/1, Divide1/2, Sum/1
  Divide1/1 -> Gain1/1
  Abs/1 -> Divide1/1
  Add1/1 -> Sum1/2
  Kd/1 -> Add1/3
  Gain1/1 -> Add/2
  Gain/1 -> Add/1
  Discrete Derivative/1 -> Gain/1
  [ResetSW] -> Discrete-Time Integrator/2

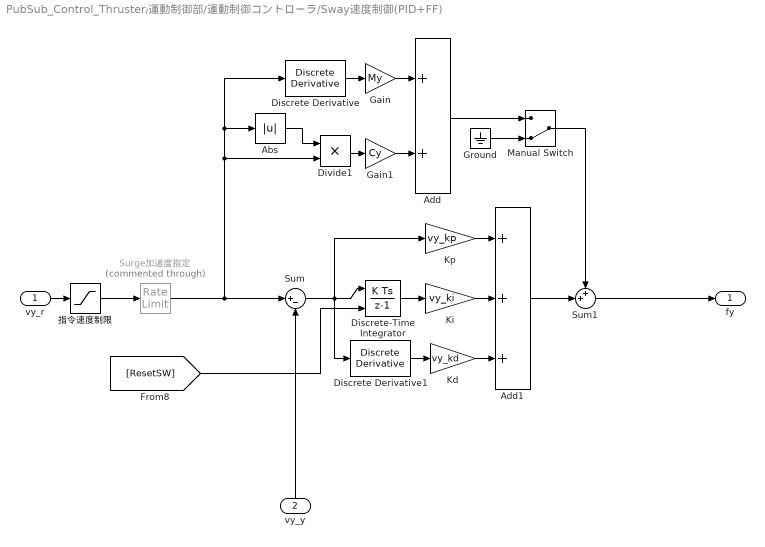
== system PubSub_Control_Thruster/運動制御部/運動制御コントローラ/Sway速度制御(PID+FF) ==
  vy_r : Inport
  vy_y : Inport  Port=2
  Abs : Abs
  Add : Sum
  Add1 : Sum  Inputs=+++
  Discrete Derivative : simulink/Discrete/Discrete Derivative  gainval=1.0  ICPrevScaledInput=0.0  InputProcessing=Inherited  OutMin=[]  OutMax=[]  OutDataType=fixdt(1, 16)  OutScaling=2^-10  DoSatur=off
  Discrete Derivative1 : simulink/Discrete/Discrete Derivative  gainval=1.0  ICPrevScaledInput=0.0  InputProcessing=Inherited  OutMin=[]  OutMax=[]  OutDataType=fixdt(1, 16)  OutScaling=2^-10  DoSatur=off
  Discrete-Time Integrator : DiscreteIntegrator  ExternalReset=rising  SampleTime=-1  ICPrevOutput=DiscIntNeverNeededParam  ICPrevScaledInput=DiscIntNeverNeededParam
  Divide1 : Product  Inputs=**
  Gain : Gain  Gain=My
  Gain1 : Gain  Gain=Cy
  Ground : Ground
  Kd : Gain  Gain=vy_kd
  Ki : Gain  Gain=vy_ki
  Kp : Gain  Gain=vy_kp
  Manual Switch : ManualSwitch  CurrentSetting=0
  Sum : Sum  Inputs=|+-
  Sum1 : Sum  Inputs=++|
  Surge加速度指定 : RateLimiter  Commented=through  RisingSlewLimit=0.1  FallingSlewLimit=-0.1  SampleTimeMode=inherited
  指令速度制限 : Saturate  UpperLimit=0.1  LowerLimit=-0.1
  fy : Outport
  wires:
  Manual Switch/1 -> Sum1/1
  Ground/1 -> Manual Switch/2
  Add/1 -> Manual Switch/1
  vy_y/1 -> Sum/2
  vy_r/1 -> 指令速度制限/1
  Kp/1 -> Add1/1
  Sum1/1 -> fy/1
  Discrete-Time Integrator/1 -> Ki/1
  Ki/1 -> Add1/2
  Sum/1 -> Discrete-Time Integrator/1, Kp/1, Discrete Derivative1/1
  Discrete Derivative1/1 -> Kd/1
  Surge加速度指定/1 -> Abs/1, Discrete Derivative/1, Divide1/2, Sum/1
  Divide1/1 -> Gain1/1
  Abs/1 -> Divide1/1
  Add1/1 -> Sum1/2
  Kd/1 -> Add1/3
  指令速度制限/1 -> Surge加速度指定/1
  Gain1/1 -> Add/2
  Gain/1 -> Add/1
  Discrete Derivative/1 -> Gain/1
  [ResetSW] -> Discrete-Time Integrator/2

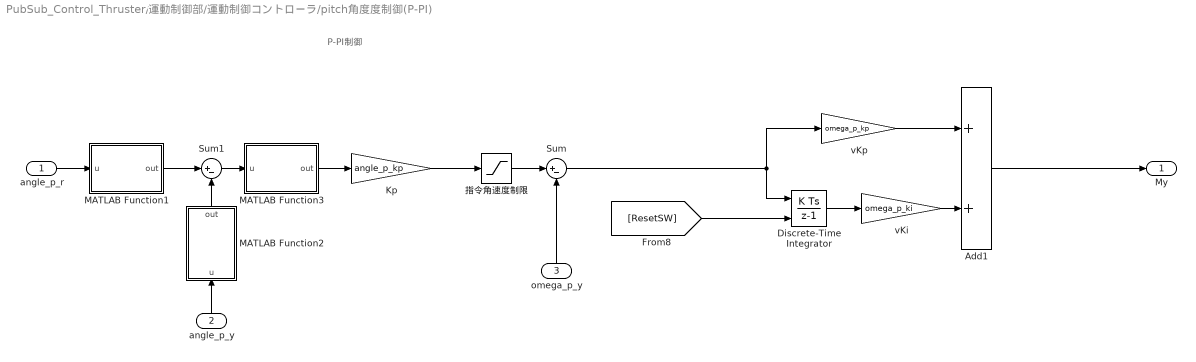
== system PubSub_Control_Thruster/運動制御部/運動制御コントローラ/pitch角度度制御(P-PI) ==
  note: P-PI制御
  angle_p_r : Inport
  angle_p_y : Inport  Port=2
  omega_p_y : Inport  Port=3
  Add1 : Sum
  Discrete-Time Integrator : DiscreteIntegrator  ExternalReset=rising  SampleTime=-1  ICPrevOutput=DiscIntNeverNeededParam  ICPrevScaledInput=DiscIntNeverNeededParam
  Kp : Gain  Gain=angle_p_kp
  MATLAB Function1 : MATLAB Function  TreatAsAtomicUnit=on
  MATLAB Function2 : MATLAB Function  TreatAsAtomicUnit=on
  MATLAB Function3 : MATLAB Function  TreatAsAtomicUnit=on
  Sum : Sum  Inputs=|+-
  Sum1 : Sum  Inputs=|+-
  vKi : Gain  Gain=omega_p_ki
  vKp : Gain  Gain=omega_p_kp
  指令角速度制限 : Saturate  UpperLimit=30  LowerLimit=-30
  My : Outport
  wires:
  MATLAB Function3/1(out) -> Kp/1
  MATLAB Function2/1(out) -> Sum1/2
  MATLAB Function1/1(out) -> Sum1/1
  Kp/1 -> 指令角速度制限/1
  Sum1/1 -> MATLAB Function3/1(u)
  angle_p_r/1 -> MATLAB Function1/1(u)
  angle_p_y/1 -> MATLAB Function2/1(u)
  vKp/1 -> Add1/1
  vKi/1 -> Add1/2
  omega_p_y/1 -> Sum/2
  Add1/1 -> My/1
  Discrete-Time Integrator/1 -> vKi/1
  Sum/1 -> Discrete-Time Integrator/1, vKp/1
  指令角速度制限/1 -> Sum/1
  [ResetSW] -> Discrete-Time Integrator/2

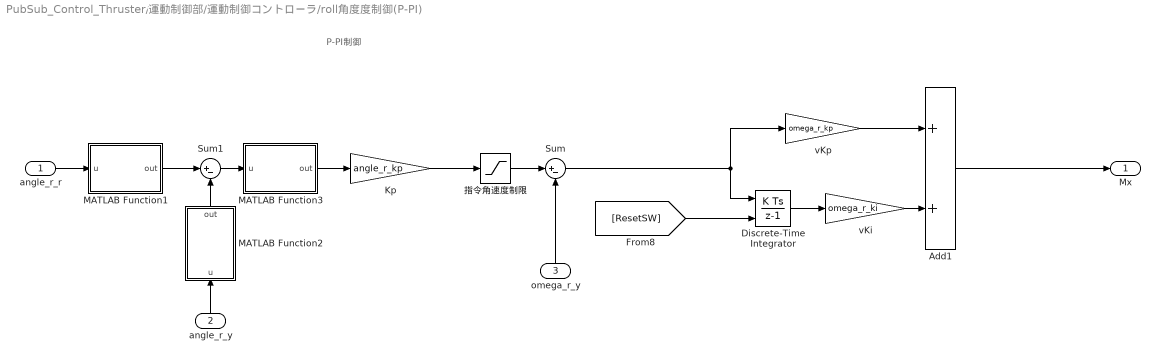
== system PubSub_Control_Thruster/運動制御部/運動制御コントローラ/roll角度度制御(P-PI) ==
  note: P-PI制御
  angle_r_r : Inport
  angle_r_y : Inport  Port=2
  omega_r_y : Inport  Port=3
  Add1 : Sum
  Discrete-Time Integrator : DiscreteIntegrator  ExternalReset=rising  SampleTime=-1  ICPrevOutput=DiscIntNeverNeededParam  ICPrevScaledInput=DiscIntNeverNeededParam
  Kp : Gain  Gain=angle_r_kp
  MATLAB Function1 : MATLAB Function  TreatAsAtomicUnit=on
  MATLAB Function2 : MATLAB Function  TreatAsAtomicUnit=on
  MATLAB Function3 : MATLAB Function  TreatAsAtomicUnit=on
  Sum : Sum  Inputs=|+-
  Sum1 : Sum  Inputs=|+-
  vKi : Gain  Gain=omega_r_ki
  vKp : Gain  Gain=omega_r_kp
  指令角速度制限 : Saturate  UpperLimit=30  LowerLimit=-30
  Mx : Outport
  wires:
  MATLAB Function3/1(out) -> Kp/1
  MATLAB Function2/1(out) -> Sum1/2
  MATLAB Function1/1(out) -> Sum1/1
  Kp/1 -> 指令角速度制限/1
  Sum1/1 -> MATLAB Function3/1(u)
  angle_r_r/1 -> MATLAB Function1/1(u)
  angle_r_y/1 -> MATLAB Function2/1(u)
  vKp/1 -> Add1/1
  vKi/1 -> Add1/2
  omega_r_y/1 -> Sum/2
  Add1/1 -> Mx/1
  Discrete-Time Integrator/1 -> vKi/1
  Sum/1 -> Discrete-Time Integrator/1, vKp/1
  指令角速度制限/1 -> Sum/1
  [ResetSW] -> Discrete-Time Integrator/2

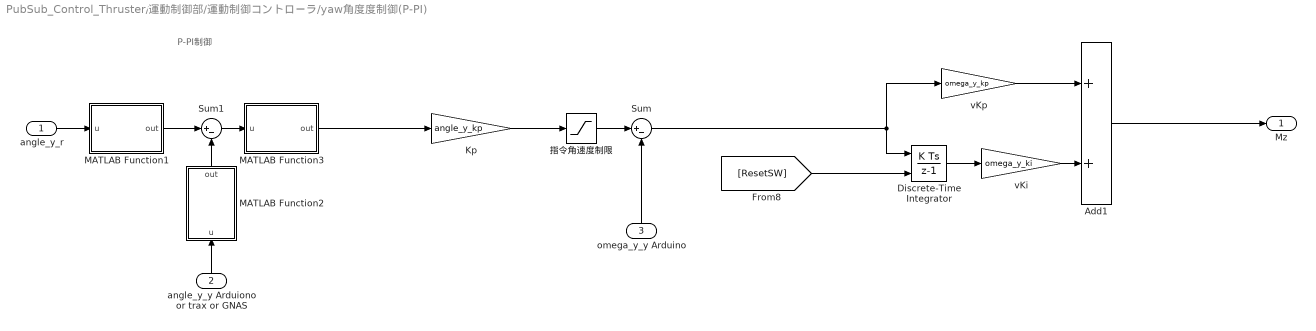
== system PubSub_Control_Thruster/運動制御部/運動制御コントローラ/yaw角度度制御(P-PI) ==
  note: P-PI制御
  angle_y_r : Inport
  angle_y_y Arduiono or trax or GNAS : Inport  Port=2
  omega_y_y Arduino : Inport  Port=3
  Add1 : Sum
  Discrete-Time Integrator : DiscreteIntegrator  ExternalReset=rising  SampleTime=-1  ICPrevOutput=DiscIntNeverNeededParam  ICPrevScaledInput=DiscIntNeverNeededParam
  Kp : Gain  Gain=angle_y_kp
  MATLAB Function1 : MATLAB Function  TreatAsAtomicUnit=on
  MATLAB Function2 : MATLAB Function  TreatAsAtomicUnit=on
  MATLAB Function3 : MATLAB Function  TreatAsAtomicUnit=on
  Sum : Sum  Inputs=|+-
  Sum1 : Sum  Inputs=|+-
  vKi : Gain  Gain=omega_y_ki
  vKp : Gain  Gain=omega_y_kp
  指令角速度制限 : Saturate  UpperLimit=30  LowerLimit=-30
  Mz : Outport
  wires:
  Kp/1 -> 指令角速度制限/1
  MATLAB Function3/1(out) -> Kp/1
  Sum1/1 -> MATLAB Function3/1(u)
  MATLAB Function2/1(out) -> Sum1/2
  MATLAB Function1/1(out) -> Sum1/1
  angle_y_r/1 -> MATLAB Function1/1(u)
  angle_y_y Arduiono or trax or GNAS/1 -> MATLAB Function2/1(u)
  vKp/1 -> Add1/1
  vKi/1 -> Add1/2
  omega_y_y Arduino/1 -> Sum/2
  Add1/1 -> Mz/1
  Discrete-Time Integrator/1 -> vKi/1
  Sum/1 -> vKp/1, Discrete-Time Integrator/1
  指令角速度制限/1 -> Sum/1
  [ResetSW] -> Discrete-Time Integrator/2

== matlab function PubSub_Control_Thruster/SaberTooth/STコマンド計算_ST1_1 ==
  data: u input; Command output
function Command = fcn(u)
% 入力の符号を判定し、コマンドを出力する関数
% 入力  操作量
% 出力  コマンド
% 
% 備考  Sabertoothのコマンドは　0：正転　1;反転
%       要仕様書確認

if 0 <= sign(u) %入力が0以上の場合
    Command = 0;
else
    Command = 1;
end

== matlab function PubSub_Control_Thruster/SaberTooth/STコマンド計算_ST1_2 ==
  data: u input; Command output
function Command = fcn(u)
% 入力の符号を判定し、コマンドを出力する関数
% 入力  操作量
% 出力  コマンド
% 
% 備考  Sabertoothのコマンドは　0：正転　1;反転
%       要仕様書確認

if 0 <= sign(u) %入力が0以上の場合
    Command = 4;
else
    Command = 5;
end

== matlab function PubSub_Control_Thruster/SaberTooth/STコマンド計算_ST2_1 ==
  data: u input; Command output
function Command = fcn(u)
% 入力の符号を判定し、コマンドを出力する関数
% 入力  操作量
% 出力  コマンド
% 
% 備考  Sabertoothのコマンドは　0：正転　1;反転
%       要仕様書確認

if 0 <= sign(u) %入力が0以上の場合
    Command = 0;
else
    Command = 1;
end

== matlab function PubSub_Control_Thruster/SaberTooth/STコマンド計算_ST2_2 ==
  data: u input; Command output
function Command = fcn(u)
% 入力の符号を判定し、コマンドを出力する関数
% 入力  操作量
% 出力  コマンド
% 
% 備考  Sabertoothのコマンドは　0：正転　1;反転
%       要仕様書確認

if 0 <= sign(u) %入力が0以上の場合
    Command = 4;
else
    Command = 5;
end

== matlab function PubSub_Control_Thruster/SaberTooth/STコマンド計算_ST3_1 ==
  data: u input; Command output
function Command = fcn(u)
% 入力の符号を判定し、コマンドを出力する関数
% 入力  操作量
% 出力  コマンド
% 
% 備考  Sabertoothのコマンドは　0：正転　1;反転
%       要仕様書確認

if 0 <= sign(u) %入力が0以上の場合
    Command = 0;
else
    Command = 1;
end

== matlab function PubSub_Control_Thruster/SaberTooth/STコマンド計算_ST3_2 ==
  data: u input; Command output
function Command = fcn(u)
% 入力の符号を判定し、コマンドを出力する関数
% 入力  操作量
% 出力  コマンド
% 
% 備考  Sabertoothのコマンドは　0：正転　1;反転
%       要仕様書確認

if 0 <= sign(u) %入力が0以上の場合
    Command = 4;
else
    Command = 5;
end

== stateflow chart PubSub_Control_Thruster/運動制御部/位置追従制御 ==
  state WP_MOVE
    %目標地点への航行
    en:
    offset = zeros(6,1);
    state move
      %DaryaBird速度指令
      en:
      flag_goal = 0;
      flag_goal_out = 0;
      flag_surge = 0;
      du:
      pos_out2 = pos_out - offset;%オフセットの追加
      [velo_in, flag_goal, flag_surge] = line_track(pos_ref,pos_out2,velo_out);
      exit:
      pos_ref_now=pos_ref;
      state surge_on
        du:
        velo_ref = [0.1; velo_in(2); velo_in(3); 0; 0; velo_in(4)];
        %velo_in2 = [0.2; velo_in(2); velo_in(3); velo_in(4)];
      state surge_off
        du:
        velo_ref = [0; velo_in(2); velo_in(3); 0; 0; velo_in(4)];
      state [velo_in,flag_goal,flag_surge] = line_track(pos_ref,pos_out,velo_out) [function]
      surge_on -> surge_off : [flag_surge == 0]
      surge_off -> surge_on : [flag_surge == 1]
      (default) -> surge_off
    state goal
      %到達フラグ出力
      en:;
      enZ = pos_out(3);
      enHead = pos_out(6);
      pos_ref_now=pos_ref;
      du:
      flag_goal_out = 1
      velo_ref = [0; 0; enZ; 0; 0; enHead];
    state pos_RESET
      %現在位置を原点にオフセットをかける
      en:
      enZ = pos_out(3);
      enHead = pos_out(6);
      du:
      offset = [pos_out(1);pos_out(2); 0; 0; 0; 0];
      velo_ref = [0; 0; enZ; 0; 0; enHead];
    (default) -> move
    move -> goal [order 1] : [flag_goal == 1]
    goal -> move : [pos_ref_now(1) ~= pos_ref(1) || pos_ref_now(2) ~= pos_ref(2) || pos_ref_now(3) ~= pos_ref(3) || pos_ref_now(6) ~= pos_ref(6)]
    pos_RESET -> move : [pos_reset == 0]
    move -> pos_RESET [order 2] : [pos_reset == 1]
  (default) -> WP_MOVE
  data: velo_in function_output double size=4; flag_goal function_output double size=1; flag_surge function_output double size=1; pos_ref function_input double size=6; pos_out function_input double size=6; velo_out function_input double size=6; velo_ref output double size=6; pos_reset input double size=1; pos_ref input double size=6; velo_out input double size=6; velo_in local double size=4; flag_goal local double; next_pos local; waypoint local double size=[100 4]; i local; pointnum local; flag_reach local double size=1; flag_surge local double size=1; velo_in_wosurge local double size=3; load_pos local; enZ local; enYaw local; pos_out input; pos_next local double size=4; wp_num_now local double size=1; pos_load local double size=[1 4]; waypoints local double size=[100 4 10]; i2 local; wp_now local double size=[100 4]; waypoints_load local double size=[1000 4]; flag_goal_out output; pos_ref_now local; offset local; pos_out2 local; enHead local

== matlab function PubSub_Control_Thruster/運動制御部/位置追従制御/WP_MOVE.move.line_track/MATLAB Function ==
  data: delta_l input; delta_w output; theta input
function delta_w = rotation_mat(delta_l,theta)
%#codegen
R = [   cosd(theta) sind(theta);
       -sind(theta) cosd(theta)];
delta_w = R * [delta_l(1); delta_l(2)];

== matlab function PubSub_Control_Thruster/運動制御部/位置追従制御/WP_MOVE.move.line_track/MATLAB Function1 ==
  data: delta_l input; delta_w output; theta input
function delta_w = rotation_mat2(delta_l,theta)
%#codegen

R = [   cosd(theta) sind(theta);
       -sind(theta) cosd(theta)];
delta_w = R * [0; delta_l(2)];
if abs(delta_w(1)) > 0.05
 delta_w = delta_w ./ sqrt(delta_l(2)^2) .* 0.05;
end

== matlab function PubSub_Control_Thruster/運動制御部/位置追従制御/WP_MOVE.move.line_track/Surge_on//offフラグ生成 ==
  data: delta_y input; flag_surge output; delta_z input; delta_yaw input; velo_yaw input
function flag_surge = rotation_mat(delta_y,delta_z,delta_yaw,velo_yaw)
%#codegen
if  abs(delta_y) < 0.3 && abs(delta_z) < 0.3 && abs(delta_yaw) < 10 && abs(velo_yaw) <10
    flag_surge = 1;
else
    flag_surge = 0;
end

== matlab function PubSub_Control_Thruster/運動制御部/位置追従制御/WP_MOVE.move.line_track/theta2delta_theta/MATLAB Function ==
  data: theta_in input; theta_out output
function theta_out = conv_theta(theta_in)%#codegen
if theta_in > 180
    theta_out = theta_in -360;
elseif theta_in < -180
    theta_out = theta_in + 360;
else
    theta_out = theta_in;
end

== matlab function PubSub_Control_Thruster/運動制御部/位置追従制御/WP_MOVE.move.line_track/theta2delta_theta/MATLAB Function1 ==
  data: theta_in input; theta_out output
function theta_out = conv_theta(theta_in)%#codegen
if theta_in > 180
    theta_out = theta_in -360;
elseif theta_in < -180
    theta_out = theta_in + 360;
else
    theta_out = theta_in;
end

== matlab function PubSub_Control_Thruster/運動制御部/位置追従制御/WP_MOVE.move.line_track/theta2delta_theta/MATLAB Function2 ==
  data: theta_in input; theta_out output
function theta_out = conv_theta(theta_in)%#codegen
if theta_in > 180
    theta_out = theta_in -360;
elseif theta_in < -180
    theta_out = theta_in + 360;
else
    theta_out = theta_in;
end

== matlab function PubSub_Control_Thruster/運動制御部/位置追従制御/WP_MOVE.move.line_track/目標点到達フラグ生成 ==
  data: delta input; flag_reach output; velo_yaw input
function flag_reach = rotation_mat(delta,velo_yaw)
%#codegen
if  delta(1) < 0 &&  abs(delta(2)) < 0.3 && abs(delta(3)) < 0.3 %&& abs(delta(4)) < 10 && abs(velo_yaw) < 10
    flag_reach = 1;
else
    flag_reach = 0;
end

== matlab function PubSub_Control_Thruster/運動制御部/運動制御コントローラ/pitch角度度制御(P-PI)/MATLAB Function1 ==
  data: u input; out output
function out = fcn(u)
%#codegen
if u > 180 
   out = u - 360;
elseif u < -180
   out = u + 360;
else
   out= u;
end
end

== matlab function PubSub_Control_Thruster/運動制御部/運動制御コントローラ/pitch角度度制御(P-PI)/MATLAB Function2 ==
  data: u input; out output
function out = fcn(u)
%#codegen
if u > 180 
   out = u - 360;
elseif u < -180
   out = u + 360;
else
   out= u;
end
end

== matlab function PubSub_Control_Thruster/運動制御部/運動制御コントローラ/pitch角度度制御(P-PI)/MATLAB Function3 ==
  data: u input; out output
function out = fcn(u)
%#codegen
if u > 180 
   out = u - 360;
elseif u < -180
   out = u + 360;
else
   out= u;
end
end

== matlab function PubSub_Control_Thruster/運動制御部/運動制御コントローラ/roll角度度制御(P-PI)/MATLAB Function1 ==
  data: u input; out output
function out = fcn(u)
%#codegen
if u > 180 
   out = u - 360;
elseif u < -180
   out = u + 360;
else
   out= u;
end
end

== matlab function PubSub_Control_Thruster/運動制御部/運動制御コントローラ/roll角度度制御(P-PI)/MATLAB Function2 ==
  data: u input; out output
function out = fcn(u)
%#codegen
if u > 180 
   out = u - 360;
elseif u < -180
   out = u + 360;
else
   out= u;
end
end

== matlab function PubSub_Control_Thruster/運動制御部/運動制御コントローラ/roll角度度制御(P-PI)/MATLAB Function3 ==
  data: u input; out output
function out = fcn(u)
%#codegen
if u > 180 
   out = u - 360;
elseif u < -180
   out = u + 360;
else
   out= u;
end
end

== matlab function PubSub_Control_Thruster/運動制御部/運動制御コントローラ/yaw角度度制御(P-PI)/MATLAB Function1 ==
  data: u input; out output
function out = fcn(u)
%#codegen
if u > 180 
   out = u - 360;
elseif u < -180
   out = u + 360;
else
   out= u;
end
end

== matlab function PubSub_Control_Thruster/運動制御部/運動制御コントローラ/yaw角度度制御(P-PI)/MATLAB Function2 ==
  data: u input; out output
function out = fcn(u)
%#codegen
if u > 180 
   out = u - 360;
elseif u < -180
   out = u + 360;
else
   out= u;
end
end

== matlab function PubSub_Control_Thruster/運動制御部/運動制御コントローラ/yaw角度度制御(P-PI)/MATLAB Function3 ==
  data: u input; out output
function out = fcn(u)
%#codegen
if u > 180 
   out = u - 360;
elseif u < -180
   out = u + 360;
else
   out= u;
end
end
